simulink model "JK_Flip_Flop"  (R2020a)
settings: Solver=VariableStepAuto  StartTime=0.0  StopTime=10.0  RelTol=1e-3
libraries: simulink_extras x1
settings Model: Creator=ashwin  LastModifiedBy=ashwin

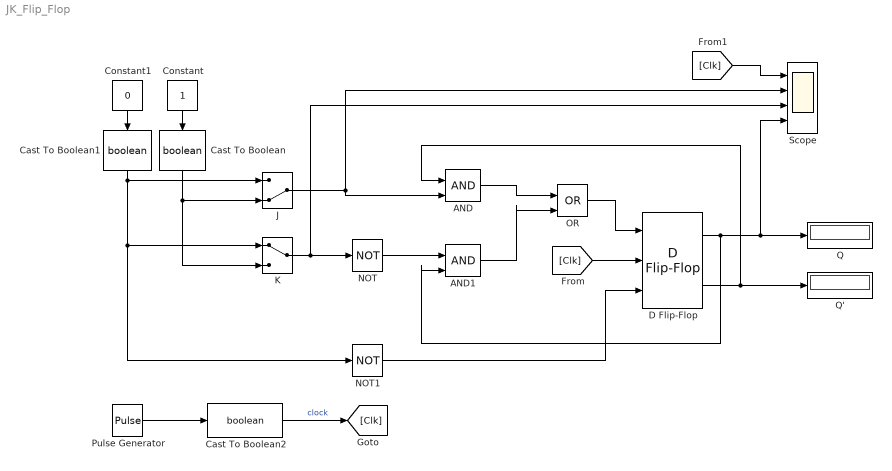
== system JK_Flip_Flop ==
  AND : Logic  IconShape=distinctive  AllPortsSameDT=off  OutDataTypeStr=boolean
  AND1 : Logic  IconShape=distinctive  AllPortsSameDT=off  OutDataTypeStr=boolean
  Cast To Boolean : DataTypeConversion  OutDataTypeStr=boolean
  Cast To Boolean1 : DataTypeConversion  OutDataTypeStr=boolean
  Cast To Boolean2 : DataTypeConversion  OutDataTypeStr=boolean
  Constant : Constant
  Constant1 : Constant  Value=0
  D Flip-Flop : simulink_extras/Flip Flops/D Flip-Flop
  J : ManualSwitch  CurrentSetting=0
  K : ManualSwitch
  NOT : Logic  Operator=NOT  IconShape=distinctive  AllPortsSameDT=off  OutDataTypeStr=boolean
  NOT1 : Logic  Operator=NOT  IconShape=distinctive  AllPortsSameDT=off  OutDataTypeStr=boolean
  OR : Logic  Operator=OR  IconShape=distinctive  AllPortsSameDT=off  OutDataTypeStr=boolean
  Pulse Generator : DiscretePulseGenerator  PulseType=Time based  PulseWidth=50
  Q : Display
  Q' : Display
  Scope : Scope  NumInputPorts=4
  wires:
  OR/1 -> D Flip-Flop/1
  AND/1 -> OR/1
  AND1/1 -> OR/2
  NOT/1 -> AND1/1
  [Clk] -> D Flip-Flop/2
  Pulse Generator/1 -> Cast To Boolean2/1
  K/1 -> Scope/3, NOT/1
  J/1 -> Scope/2, AND/2
  Constant1/1 -> Cast To Boolean1/1
  Constant/1 -> Cast To Boolean/1
  D Flip-Flop/2 -> AND/1, Q'/1
  D Flip-Flop/1 -> AND1/2, Scope/4, Q/1
  Cast To Boolean/1 -> J/2, K/2
  Cast To Boolean1/1 -> J/1, NOT1/1, K/1
  Cast To Boolean2/1 -> [Clk]  "clock"
  NOT1/1 -> D Flip-Flop/3
  [Clk] -> Scope/1
